simulink model "Sim_cont_LQ"  (Simulink 7.5)
settings: Solver=ode3  StartTime=0.0  StopTime=10.0  FixedStep=0.02  RelTol=1e-3
undefined symbols (not defined in the file): Adr, Bdr, Cdr, Ddr, Kff, Kglob
libraries: simulink x2
settings Model: Creator=fclaveau  LastModifiedBy=fclaveau

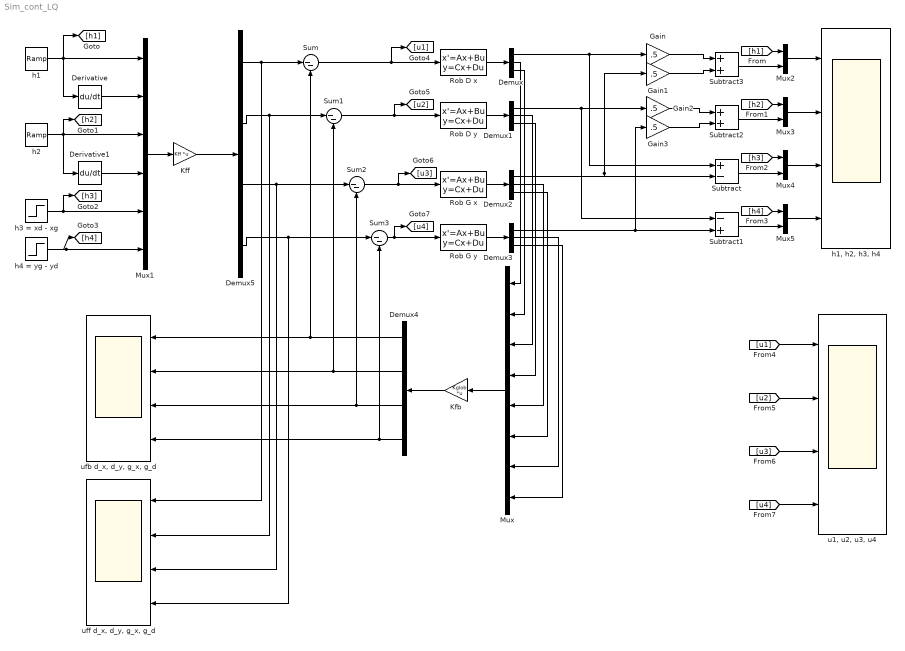
== system Sim_cont_LQ ==
  Demux{,1..3} (4 alike) : Demux  Outputs=3
  Demux4 : Demux
  Demux5 : Demux
  Derivative : Derivative
  Derivative1 : Derivative
  Gain{,1..3} (4 alike) : Gain  Gain=.5  ParameterDataType=fixdt(1, 16)  ParameterScaling=2^0  OutDataType=fixdt(1, 16)  OutScaling=2^0
  Kfb : Gain  Gain=Kglob  Multiplication=Matrix(K*u)  ParameterDataType=fixdt(1, 16)  ParameterScaling=2^0  OutDataType=fixdt(1, 16)  OutScaling=2^0
  Kff : Gain  Gain=Kff  Multiplication=Matrix(K*u)  ParameterDataType=fixdt(1, 16)  ParameterScaling=2^0  OutDataType=fixdt(1, 16)  OutScaling=2^0
  Mux : Mux  Inputs=8
  Mux1 : Mux  Inputs=6
  Mux{2..5} (4 alike) : Mux  Inputs=2
  "Rob D x " : StateSpace  A=Adr  B=Bdr  C=Cdr  D=Ddr
  Rob D y : StateSpace  A=Adr  B=Bdr  C=Cdr  D=Ddr
  Rob G x : StateSpace  A=Adr  B=Bdr  C=Cdr  D=Ddr
  Rob G y : StateSpace  A=Adr  B=Bdr  C=Cdr  D=Ddr
  Subtract : Sum  Inputs=+-  OutDataType=fixdt(1, 16)  OutScaling=2^-10
  Subtract1 : Sum  Inputs=-+  OutDataType=fixdt(1, 16)  OutScaling=2^-10
  Subtract2 : Sum  OutDataType=fixdt(1, 16)  OutScaling=2^-10
  Subtract3 : Sum  OutDataType=fixdt(1, 16)  OutScaling=2^-10
  Sum{,1..3} (4 alike) : Sum  Inputs=|--  OutDataType=fixdt(1, 16)  OutScaling=2^0
  h1 : simulink/Sources/Ramp  SystemSampleTime=-1  slope=1  start=1  X0=0
  "h1, h2, h3, h4" : Scope  NumInputPorts=4
      settings: YMin=-5~-5~-5~-5  YMax=5~5~5~5
  h2 : simulink/Sources/Ramp  SystemSampleTime=-1  slope=1  start=3  X0=0
  h3 = xd - xg : Step  Time=5  SampleTime=0
  h4 = yg - yd : Step  Time=7  SampleTime=0
  "u1, u2, u3, u4" : Scope  NumInputPorts=4
      settings: YMin=-5~-5~-5~-5  YMax=5~5~5~5  SaveName=ScopeData3
  "ufb d_x, d_y, g_x, g_d" : Scope  NumInputPorts=4
      settings: YMin=-5~-5~-5~-5  YMax=5~5~5~5
  "uff d_x, d_y, g_x, g_d" : Scope  NumInputPorts=4
      settings: YMin=-5~-5~-5~-5  YMax=5~5~5~5  SaveName=ScopeData2
  wires:
  Gain/1 -> Subtract3/1
  Gain1/1 -> Subtract3/2
  "Rob D x "/1 -> Demux/1
  Rob D y/1 -> Demux1/1
  Rob G x/1 -> Demux2/1
  Rob G y/1 -> Demux3/1
  Demux/1 -> Gain/1, Subtract/1
  Demux2/1 -> Gain1/1, Subtract/2
  Gain2/1 -> Subtract2/1
  Gain3/1 -> Subtract2/2
  Demux1/1 -> Gain2/1, Subtract1/1
  Demux3/1 -> Gain3/1, Subtract1/2
  Mux/1 -> Kfb/1
  Kfb/1 -> Demux4/1
  Demux4/1 -> Sum/2, "ufb d_x, d_y, g_x, g_d"/1
  Sum/1 -> [u1], "Rob D x "/1
  Sum1/1 -> [u2], Rob D y/1
  Demux4/2 -> Sum1/2, "ufb d_x, d_y, g_x, g_d"/2
  Sum2/1 -> [u3], Rob G x/1
  Demux4/3 -> Sum2/2, "ufb d_x, d_y, g_x, g_d"/3
  Sum3/1 -> [u4], Rob G y/1
  Demux4/4 -> Sum3/2, "ufb d_x, d_y, g_x, g_d"/4
  Demux5/1 -> Sum/1, "uff d_x, d_y, g_x, g_d"/1
  Demux5/4 -> Sum3/1, "uff d_x, d_y, g_x, g_d"/4
  Demux5/2 -> Sum1/1, "uff d_x, d_y, g_x, g_d"/2
  Demux5/3 -> Sum2/1, "uff d_x, d_y, g_x, g_d"/3
  Kff/1 -> Demux5/1
  Mux1/1 -> Kff/1
  h3 = xd - xg/1 -> Mux1/5, [h3]
  h4 = yg - yd/1 -> Mux1/6, [h4]
  h2/1 -> Mux1/3, Derivative1/1, [h2]
  h1/1 -> Mux1/1, Derivative/1, [h1]
  Derivative/1 -> Mux1/2
  Derivative1/1 -> Mux1/4
  Mux2/1 -> "h1, h2, h3, h4"/1
  Mux3/1 -> "h1, h2, h3, h4"/2
  Mux4/1 -> "h1, h2, h3, h4"/3
  Mux5/1 -> "h1, h2, h3, h4"/4
  Subtract3/1 -> Mux2/2
  Subtract2/1 -> Mux3/2
  Subtract/1 -> Mux4/2
  Subtract1/1 -> Mux5/2
  [h1] -> Mux2/1
  [h2] -> Mux3/1
  [h3] -> Mux4/1
  [h4] -> Mux5/1
  [u1] -> "u1, u2, u3, u4"/1
  [u2] -> "u1, u2, u3, u4"/2
  [u3] -> "u1, u2, u3, u4"/3
  [u4] -> "u1, u2, u3, u4"/4
  Demux/2 -> Mux/1
  Demux/3 -> Mux/2
  Demux1/2 -> Mux/3
  Demux1/3 -> Mux/4
  Demux2/2 -> Mux/5
  Demux2/3 -> Mux/6
  Demux3/2 -> Mux/7
  Demux3/3 -> Mux/8
